simulink model "EPS_Dynamic_Model_Trinh_Tien_Long"  (R2022b)
settings: Solver=VariableStepAuto  StartTime=0.0  StopTime=8  MaxStep=0.001  RelTol=1e-3
undefined symbols (not defined in the file): Br, Bs, im, Js, km, kr, ks, m, rp, sigbuilder_block
settings Model: Creator=dangm  LastModifiedBy=ASUS
settings SolverCC: AlgebraicLoopSolver=TrustRegion
settings DebuggingCC: UnconnectedInputMsg=warning  UnconnectedOutputMsg=warning  UnconnectedLineMsg=warning  SFMachineParentedDataDiag=warning
settings ModelReferenceCC: EnableRefExpFcnMdlSchedulingChecks=on

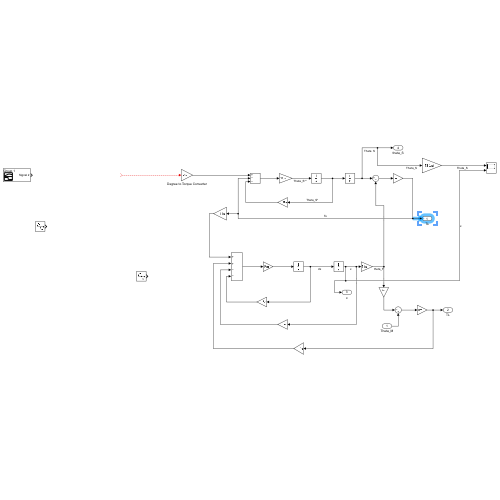
[thumbnail: Simulink's stored preview of the top-level diagram]
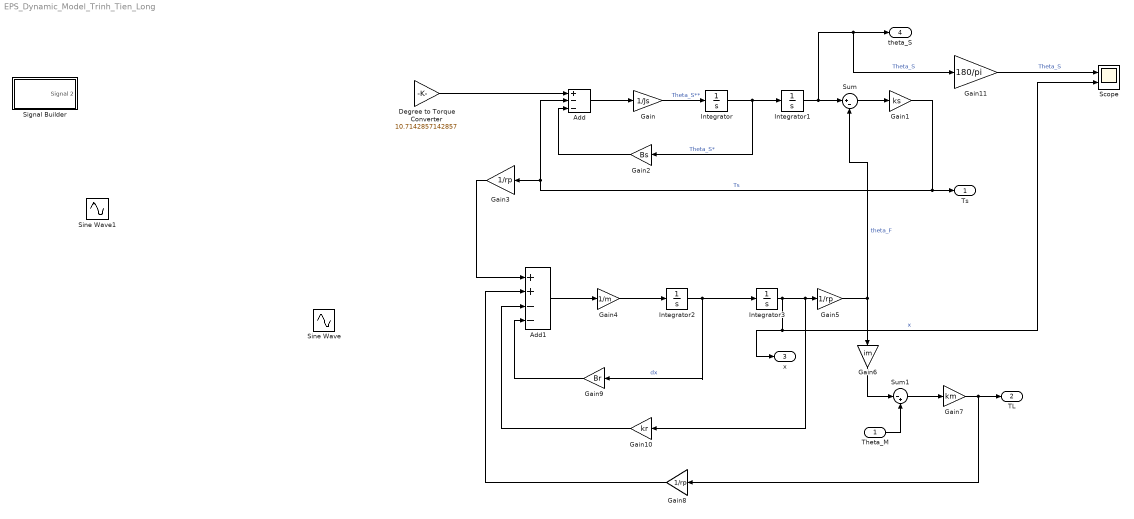
== system EPS_Dynamic_Model_Trinh_Tien_Long ==
  Theta_M : Inport
  Add : Sum  Inputs=+--
  Add1 : Sum  Inputs=++--
  Degree to Torque Converter : Gain  Gain=10.7142857142857
  Gain : Gain  Gain=1/Js
  Gain1 : Gain  Gain=ks
  Gain10 : Gain  Gain=kr
  Gain11 : Gain  Gain=180/pi
  Gain2 : Gain  Gain=Bs
  Gain3 : Gain  Gain=1/rp
  Gain4 : Gain  Gain=1/m
  Gain5 : Gain  Gain=1/rp
  Gain6 : Gain  Gain=im
  Gain7 : Gain  Gain=km
  Gain8 : Gain  Gain=1/rp
  Gain9 : Gain  Gain=Br
  Integrator{,1..3} (4 alike) : Integrator
  Scope : Scope  NumInputPorts=2
  Signal Builder : Subsystem  Tag=STV Subsys  LoadFcn=sigbuilder_block('load');  StartFcn=sigbuilder_block('start');  StopFcn=sigbuilder_block('stop');  ClipboardFcn=sigbuilder_block('clipboard');  mask(Sigbuilder block){tuvar=[0:10]}
      mask help: Simulink:masks:SigbuilderBlock_MD
      mask init:
      | if ~strcmp(get_param(bdroot(gcbh),'SimulationStatus'),'stopped') tuvar = sigbuilder_block('maskInit'); end
      settings: CopyFcn=sigbuilder_block('copy');  DeleteFcn=sigbuilder_block('delete');  ModelCloseFcn=sigbuilder_block('modelClose');  PreSaveFcn=sigbuilder_block('preSave');  PauseFcn=sigbuilder_block('pause');  ContinueFcn=sigbuilder_block('continue');  NameChangeFcn=sigbuilder_block('namechange');  OpenFcn=sigbuilder_block('open',[404 117.5 550.5 362.5 ]);  CloseFcn=sigbuilder_block('close');
      mask Display: plot(0, 0, 100, 100,[2, 2, 32, 32, 2], [68, 8, 8, 68, 68],[32, 2], [38, 38], [32, 19, 2],[53, 60, 44], [32, 17, 17, 2],[16, 16, 31, 31]);txt = getActiveGroup(gcbh);text(2, 100, txt,'verticalAlignment', 'top');
  Sine Wave : Sin  Amplitude=28  Frequency=2  SampleTime=0
  Sine Wave1 : Sin  Amplitude=28  SampleTime=0
  Sum : Sum  Inputs=|+-
  Sum1 : Sum  Inputs=|-+
  Ts : Outport
  "TL " : Outport  Port=2
  x : Outport  Port=3
  theta_S : Outport  Port=4
  wires:
  Add/1 -> Gain/1
  Gain/1 -> Integrator/1  "Theta_S**"
  Integrator/1 -> Gain2/1, Integrator1/1  "Theta_S*"
  Integrator1/1 -> Gain11/1, theta_S/1, Sum/1  "Theta_S"
  Sum/1 -> Gain1/1
  Gain2/1 -> Add/3
  Gain1/1 -> Add/2, Gain3/1, Ts/1  "Ts"
  Gain3/1 -> Add1/1
  Add1/1 -> Gain4/1
  Gain4/1 -> Integrator2/1
  Integrator2/1 -> Gain9/1, Integrator3/1  "dx"
  Integrator3/1 -> Scope/2, x/1, Gain10/1, Gain5/1  "x"
  Gain5/1 -> Sum/2, Gain6/1  "theta_F"
  Gain6/1 -> Sum1/1
  Sum1/1 -> Gain7/1
  Gain7/1 -> "TL "/1, Gain8/1
  Gain8/1 -> Add1/2
  Gain9/1 -> Add1/4
  Gain10/1 -> Add1/3
  Theta_M/1 -> Sum1/2
  Gain11/1 -> Scope/1  "Theta_S"
  ? -> Degree to Torque Converter/1
  Degree to Torque Converter/1 -> Add/1

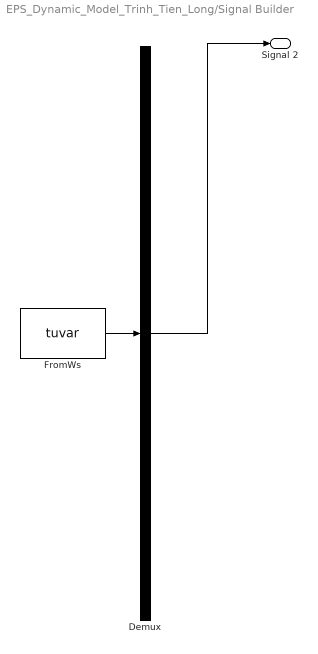
== system EPS_Dynamic_Model_Trinh_Tien_Long/Signal Builder ==
  Demux : Demux  Tag=STV Demux  Outputs=1
      settings: DisplayOption=none
  FromWs : FromWorkspace  Tag=STV FromWs  VariableName=tuvar
      SigBuilderData=|
      | common.afterFinalStr = 'Extrapolate'
      | common.sampleTime = 0
      | dataSet.timeRange = [0 10]
      | dataSet.name = 'Group 1'
      | sbobj.Groups.Name = 'Group 1'
      | sbobj.Groups.Signals.Name = 'Signal 2'
      | sbobj.Groups.Signals.XData = [0 3 3 10]
      | sbobj.Groups.Signals.YData = [0 0 5 5]
  Signal 2 : Outport  Tag=STV Outport
  wires:
  FromWs/1 -> Demux/1
  Demux/1 -> Signal 2/1
